simulink model "HSLS_Inbetriebnahme_SS21_090621"  (R2021a)
settings: Solver=FixedStepDiscrete  StartTime=0.0  StopTime=inf  FixedStep=TA  RelTol=1e-3
libraries: arduinolib x4, hdlsllib x1
settings Model: FPTRunName=Active  SimulationMode=external  SILPILModeSetting=veronly  ExtModeTrigDuration=2  Creator=The MathWorks, Inc.  LastModifiedBy=Amin Seffo
settings SolverCC: AlgebraicLoopSolver=TrustRegion
settings DataIOCC: LimitDataPoints=on  SaveFormat=Array  ReturnWorkspaceOutputs=off
settings OptimizationCC: ExpressionDepthLimit=2147483647  LifeSpan=Inf  MaxStackSize=64
settings DebuggingCC: UnderspecifiedInitializationDetection=Classic  MergeDetectMultiDrivingBlocksExec=none  FcnCallInpInsideContextMsg=warning  AllowSymbolicDim=off  StateNameClashWarn=warning  SFUnexpectedBacktrackingDiag=warning  SFNoUnconditionalDefaultTransitionDiag=warning  SFExecutionAtInitializationDiag=none  SFMachineParentedDataDiag=warning  ArithmeticOperatorsInVariantConditions=warning
settings HardwareCC: ProdBitPerPointer=32  ProdBitPerSizeT=32  ProdBitPerPtrDiffT=32  ProdLargestAtomicInteger=Long  ProdLargestAtomicFloat=Double  ProdWordSize=32  ProdHWDeviceType=ARM Compatible->ARM Cortex  UseEmbeddedCoderFeatures=off  UseSimulinkCoderFeatures=off
settings ModelReferenceCC: PropagateSignalLabelsOutOfModel=off
settings SFSimCC: SimUseLocalCustomCode=off  MATLABDynamicMemAlloc=off
settings RTWCC: SystemTargetFile=ert.tlc  HardwareBoard=Arduino Nano 33 IoT  TemplateMakefile=ert_default_tmf  RTWVerbose=off  RTWUseLocalCustomCode=off  Toolchain=Arduino ARM  BuildConfiguration=Faster Runs
settings RTWCC: CustomInitializer=|
  | /* Enable GCLK0 for the ADC
  |   GCLK->CLKCTRL.reg = GCLK_CLKCTRL_CLKEN |
  |                       GCLK_CLKCTRL_GEN_GCLK0 |
  |                       GCLK_CLKCTRL_ID_ADC;*/
  | 
  |   while (GCLK->STATUS.bit.SYNCBUSY) {};    /* Wait for bus synchronization. */
  | 
  |   while (ADC->STATUS.bit.SYNCBUSY);                  // Wait for synchronization
  | 
  |   ADC->SAMPCTRL.bit.SAMPLEN = 0x8;                  // Set max Sampling Time Length to half divided ADC clock pulse (2.66us)
  |   ADC->AVGCTRL.reg = ADC_AVGCTRL_SAMPLENUM_16 | ADC_AVGCTRL_ADJRES(4);
  |   ADC->CTRLB.reg = ADC_CTRLB_PRESCALER_DIV16 |     // Divide Clock ADC GCLK by 512 (48MHz/512 = 93.7kHz)
  |                    ADC_CTRLB_RESSEL_16BIT |          // Set the ADC resolution to 16 bits --> enable averaging mode
  |                    ADC_CTRLB_FREERUN;                // Set the ADC to free run
  |   while (ADC->STATUS.bit.SYNCBUSY);                  // Wait for synchronization
settings CodeAppCC: ForceParamTrailComments=on  OperatorAnnotations=on  StateflowObjectComments=on  MATLABSourceComments=on
settings ERTTargetCC: MultiwordLength=2048  ERTCustomFileBanners=off  SupportContinuousTime=on  SupportNonInlinedSFcns=on  RemoveResetFunc=off  SupportVariableSizeSignals=on  ModelStepFunctionPrototypeControlCompliant=off  ExtModeStaticAllocSize=1024
settings ConfigComp: CovMetricSettings=dw  CovSaveCumulativeToWorkspaceVar=on  CovSaveSingleToWorkspaceVar=on  CovExternalEMLEnable=off  CovSFcnEnable=off

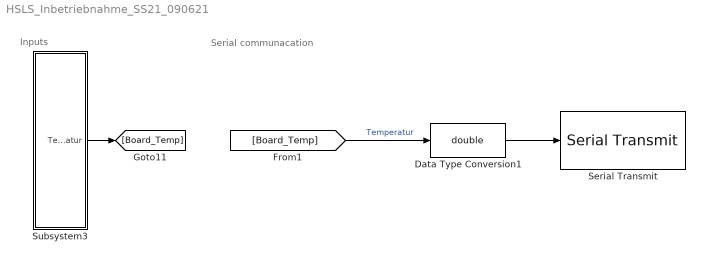
== system HSLS_Inbetriebnahme_SS21_090621 ==
  note: Serial communacation
  note: Inputs
  Data Type Conversion1 : DataTypeConversion  OutDataTypeStr=double
  Serial Transmit : arduinolib/Serial Transmit  portNumber=0  sendmode=println  sendformat=Decimal  floatprecision=2  blockPlatform=arduino
  Subsystem3 : Subsystem
  wires:
  Subsystem3/1(Temperatur) -> [Board_Temp]
  [Board_Temp] -> Data Type Conversion1/1  "Temperatur"
  Data Type Conversion1/1 -> Serial Transmit/1

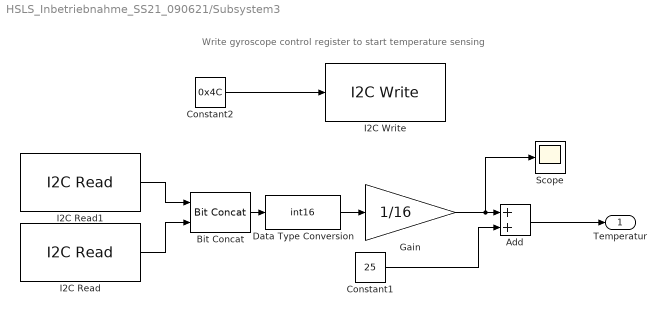
== system HSLS_Inbetriebnahme_SS21_090621/Subsystem3 ==
  note: Write gyroscope control register to start temperature sensing
  Add : Sum  AccumDataTypeStr=fixdt(1,32,15)
  Bit Concat : hdlsllib/Logic and Bit Operations/Bit Concat  numInputs=2
  Constant1 : Constant  Value=25  OutDataTypeStr=fixdt(1,32,15)  SampleTime=0.1
  Constant2 : Constant  Value=0x4C
  Data Type Conversion : DataTypeConversion  OutDataTypeStr=int16  ConvertRealWorld=Stored Integer (SI)
  Gain : Gain  Gain=1/16  OutDataTypeStr=fixdt(1,32,15)
  I2C Read : arduinolib/I2C Read  I2CModule=0  Mode=Master  SlaveAddress=0x6A  SlaveByteOrder=LittleEndian  Direction=Receiver  RegisterAddressMode=on  RegisterAddress=0x20  SlaveDataType=uint8  DataLength=1  NoAck=off  RepeatedStart=off  OutputStatus=off  blockPlatform=ARDUINO  SampleTime=0.1
      settings: SourceProductBaseCode=ARDUINO
  I2C Read1 : arduinolib/I2C Read  I2CModule=0  Mode=Master  SlaveAddress=0x6A  SlaveByteOrder=LittleEndian  Direction=Receiver  RegisterAddressMode=on  RegisterAddress=0x21  SlaveDataType=uint8  DataLength=1  NoAck=off  RepeatedStart=off  OutputStatus=off  blockPlatform=ARDUINO  SampleTime=0.1
      settings: SourceProductBaseCode=ARDUINO
  I2C Write : arduinolib/I2C Write  I2CModule=0  Mode=Master  SlaveAddress=0x6A  SlaveByteOrder=BigEndian  Direction=Transmitter  RegisterAddressMode=on  RegisterAddress=0x11  SlaveDataType=uint8  DataLength=1  NoAck=off  RepeatedStart=off  OutputStatus=off  blockPlatform=ARDUINO
      settings: SourceProductBaseCode=ARDUINO
  Scope : Scope
  Temperatur : Outport  OutDataTypeStr=fixdt(1,32,15)
  wires:
  Add/1 -> Temperatur/1
  Data Type Conversion/1 -> Gain/1
  I2C Read/1 -> Bit Concat/2
  Gain/1 -> Scope/1, Add/1
  Constant1/1 -> Add/2
  Bit Concat/1 -> Data Type Conversion/1
  I2C Read1/1 -> Bit Concat/1
  Constant2/1 -> I2C Write/1
